simulink model "adaptation_for_g"  (R2024a)
settings: Solver=VariableStepAuto  StartTime=0.0  StopTime=2000.0  MaxStep=1e-3  RelTol=1e-3
settings Model: Creator=evgenijkondratev  LastModifiedBy=evgenijkondratev

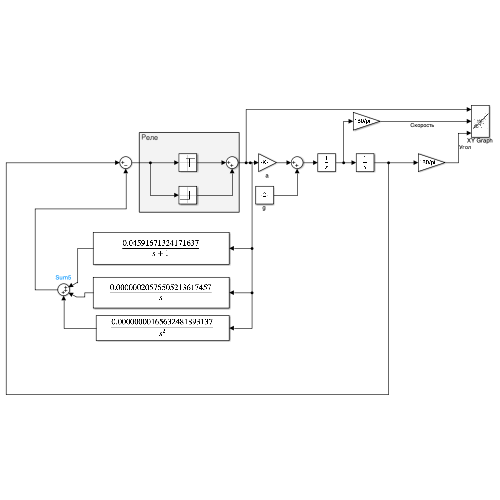
[thumbnail: Simulink's stored preview of the top-level diagram]
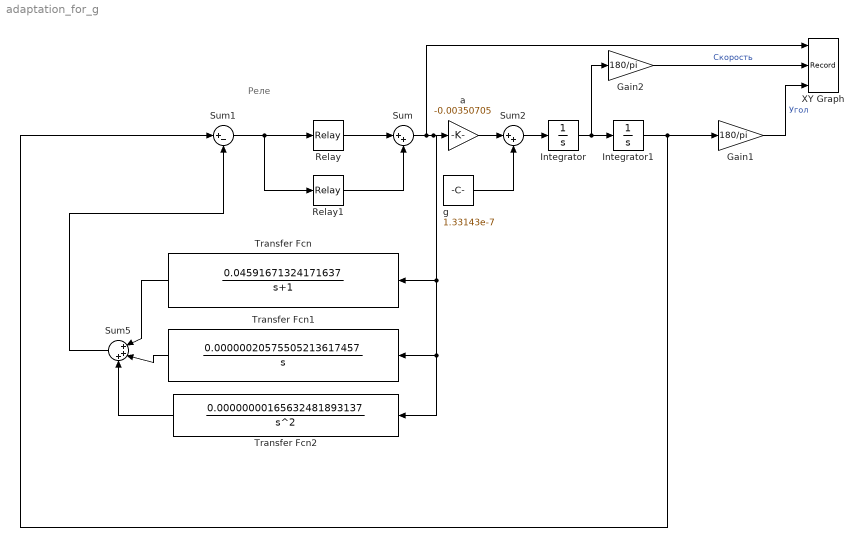
== system adaptation_for_g ==
  note: Реле
  Gain1 : Gain  Gain=180/pi
  Gain2 : Gain  Gain=180/pi
  Integrator : Integrator  InitialCondition=0.00005
  Integrator1 : Integrator  InitialCondition=0.0017593
  Relay : Relay  OnSwitchValue=0.0017593  OffSwitchValue=0.0017593-0.000351870594507
  Relay1 : Relay  OnSwitchValue=-0.0017593 + 0.000351870594507  OffSwitchValue=-0.0017593  OnOutputValue=0  OffOutputValue=-1
  Sum : Sum  Inputs=|++
  Sum1 : Sum  Inputs=|+-
  Sum2 : Sum  Inputs=|++
  Sum5 : Sum  Inputs=|+++
  Transfer Fcn : TransferFcn  Numerator=[0.04591671324171637]  Denominator=[1 1]
  Transfer Fcn1 : TransferFcn  Numerator=[0.00000020575505213617457]  Denominator=[1 0]
  Transfer Fcn2 : TransferFcn  Numerator=[0.00000000165632481893137]  Denominator=[1 0 0]
  XY Graph : Record  FileSettingsInternal="{\"entries\":[{\"content\":{\"excelSettings\":{\"content\":{},\"type\":\"Streamout.ExcelSettings\"}},\"type\":\"Streamout.FileSettingStorage\",\"uuid\":\"\"}],\"packageUris\":[\"http:\\/\\/schema.mathworks.com\\/mf0\\/streamout_blocks\\/R2020a\"],\"version\":\"1.0\"}"  Layout=[1 1]  SignalsInternal="{\"entries\":[{\"content\":{\"signals\":[{\"content\":{\"blockPath\":[],\"dimensions\":[1],\"domain\":\"\",\"lineColor\":\"#a2142f\",\"plots\":[ 1 ],\"port\":1,\"sid\":[\"\"],\"signalID\":1,\"signalName\":\"Sum\"},\"type\":\"RecordBlkView.Signal\",\"uuid\":\"\"},{\"content\":{\"blockPath\":[],\"dimensions\":[1],\"domain\":\"\",\"lineColor\":\"#0072bd\",\"lineWidth\":20,\"plots\":[ 1 ],\"port\":2,\"sid\":[\"\"],\"signalID\":2,\"signalName\":\"Скорость\"},\"type\":\"RecordBlkView.Signal\",\"uuid\":\"\"},{\"content\":{\"blockPath\":[],\"dimensions\":[1],\"domain\":\"\",\"lineColor\":\"#d95319\",\"lineWidth\":20,\"port\":3,\"sid\":[\"\"],\"signalID\":3,\"signalName\":\"Угол\"},\"type\":\"RecordBlkView.Signal\",\"uuid\":\"\"}]},\"type\":\"RecordBlkView.InputSignals\",\"uuid\":\"\"}],\"packageUris\":[\"http:\\/\\/schema.mathworks.com\\/mf0\\/streamout_blocks\\/R2020a\"],\"version\":\"1.0\"}"  VisualizationBindings="{\"xyplotplugin\":{\"info\":[{\"series\":[{\"bindingParametersList\":[{\"parameter\":\"X-Axis\",\"signalID\":1,\"signalName\":\"Sum\"},{\"parameter\":\"Y-Axis\",\"signalID\":2,\"signalName\":\"Скорость\"}],\"seriesID\":0}],\"subplotID\":1}]}}"  CompatibilityTag=XY
  a : Gain  Gain=-0.00350705
  g : Constant  Value=1.33143e-7
  wires:
  Relay/1 -> Sum/1
  Gain1/1 -> XY Graph/3  "Угол"
  Gain2/1 -> XY Graph/2  "Скорость"
  a/1 -> Sum2/1
  Integrator1/1 -> Sum1/1, Gain1/1
  Sum/1 -> Transfer Fcn2/1, Transfer Fcn1/1, Transfer Fcn/1, a/1, XY Graph/1
  Integrator/1 -> Gain2/1, Integrator1/1
  Relay1/1 -> Sum/2
  g/1 -> Sum2/2
  Sum2/1 -> Integrator/1
  Sum1/1 -> Relay/1, Relay1/1
  Transfer Fcn/1 -> Sum5/1
  Sum5/1 -> Sum1/2
  Transfer Fcn1/1 -> Sum5/2
  Transfer Fcn2/1 -> Sum5/3
